simulink model "vf_comparison"  (R2023b)
settings: Solver=VariableStepAuto  StartTime=0.0  StopTime=100  FixedStep=0.001  RelTol=1e-3
undefined symbols (not defined in the file or in its folder): J, K_r, L_m, L_s, R_s, T_r, Z_p
libraries: fuzblock x1, slpidlib x1, rllib x1, dspsrcs4 x1
settings Model: Creator=anste  LastModifiedBy=anste
settings SolverCC: ZeroCrossAlgorithm=Adaptive
settings DebuggingCC: IgnoredZcDiagnostic=none

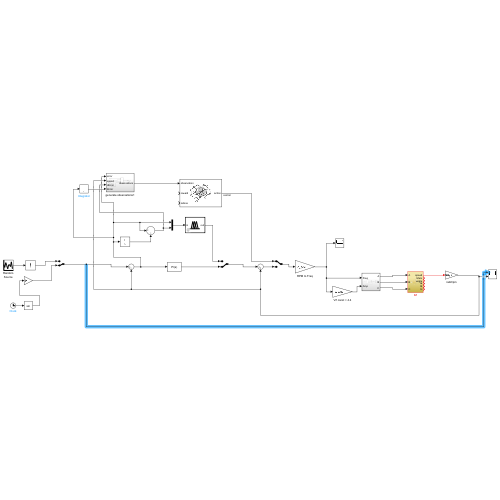
[thumbnail: Simulink's stored preview of the top-level diagram]
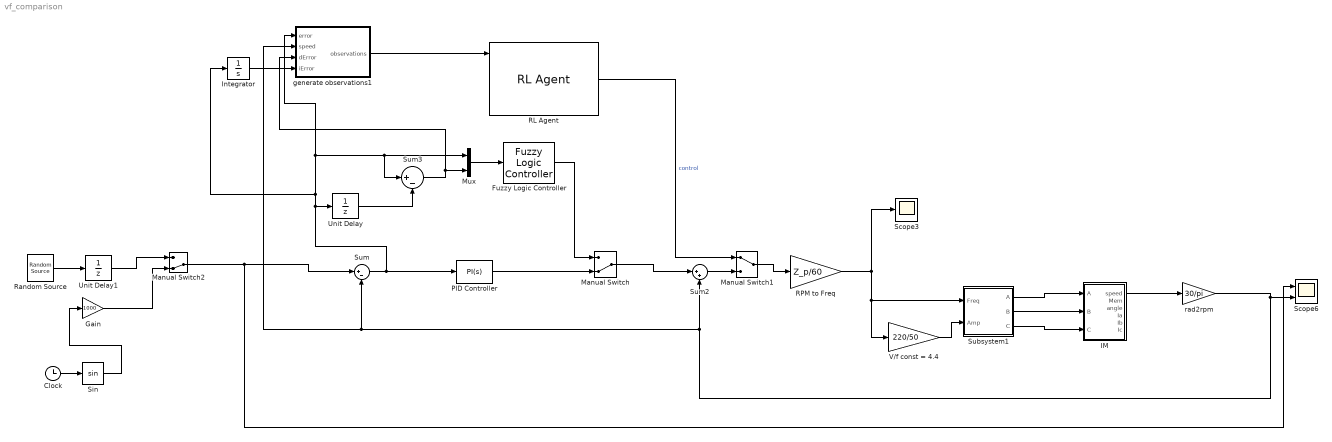
== system vf_comparison ==
  Clock : Clock
  Fuzzy Logic Controller : fuzblock/Fuzzy Logic  Controller  FIS='fuzzy35.fis'  OutputSampleNumber=101  DataType=double  FuzzifiedInputs=off  RuleFiringStrengths=off  RuleOutputs=off  AggregatedOutputs=off  SimulateUsing=Interpreted execution  OutOfRangeInputValueMessage=warning  NoRuleFiredMessage=warning  EmptyOutputFuzzySetMessage=warning
  Gain : Gain  Gain=1000
  IM : Subsystem
  Integrator : Integrator
  Manual Switch : ManualSwitch  CurrentSetting=0
  Manual Switch1 : ManualSwitch
  Manual Switch2 : ManualSwitch  CurrentSetting=0
  Mux : Mux  Inputs=2
  PID Controller : slpidlib/PID Controller  Controller=PI  Form=Parallel  TimeDomain=Continuous-time  UseExternalTs=off  SampleTime=-1  IntegratorMethod=Forward Euler  FilterMethod=Forward Euler  ControllerParametersSource=internal  P=0.42  I=0.87  UseKiTs=off  D=0.000001  N=100  UseFilter=on  TunerSelectOption=Transfer Function Based (PID Tuner App)  InitialConditionSource=internal  InitialConditionForIntegrator=0  InitialConditionForFilter=0  DifferentiatorICPrevScaledInput=0  ExternalReset=none  TrackingMode=off  Kt=1  LimitOutput=off  SatLimitsSource=internal  UpperSaturationLimit=100  LowerSaturationLimit=-100  LinearizeAsGain=on  AntiWindupMode=clamping  Kb=1  LimitIntegrator=off  UpperIntegratorSaturationLimit=inf  LowerIntegratorSaturationLimit=-inf  POutMin=[]  POutMax=[]  IOutMin=[]  IOutMax=[]  DOutMin=[]  DOutMax=[]  NOutMin=[]  NOutMax=[]  SumOutMin=[]  SumOutMax=[]  SaturationOutMin=[]  SaturationOutMax=[]  PParamMin=[]  PParamMax=[]  IParamMin=[]  IParamMax=[]  DParamMin=[]  DParamMax=[]  NParamMin=[]  NParamMax=[]  KbParamMin=[]  KbParamMax=[]  KtParamMin=[]  KtParamMax=[]  KbOutMin=[]  KbOutMax=[]  KtOutMin=[]  KtOutMax=[]  IntegratorOutMin=[]  IntegratorOutMax=[]  FilterOutMin=[]  FilterOutMax=[]  SumI1OutMin=[]  SumI1OutMax=[]  SumI2OutMin=[]  SumI2OutMax=[]  SumI3OutMin=[]  SumI3OutMax=[]  SumI4OutMin=[]  SumI4OutMax=[]  SumDOutMin=[]  SumDOutMax=[]  DifferentiatorOutMin=[]  DifferentiatorOutMax=[]  FilterDiffOutCoefMin=[]  FilterDiffOutCoefMax=[]  ReciprocalOutMin=[]  ReciprocalOutMax=[]  SumDenOutMin=[]  SumDenOutMax=[]  SumNumOutMin=[]  SumNumOutMax=[]  DivideOutMin=[]  DivideOutMax=[]  UdiffTsProdOutMin=[]  UdiffTsProdOutMax=[]  NTsProdOutMin=[]  NTsProdOutMax=[]  UintegralTsProdOutMin=[]  UintegralTsProdOutMax=[]  UngainTsProdOutMin=[]  UngainTsProdOutMax=[]  ClampingZeroOutDataTypeStr=Inherit: Inherit via back propagation  ClampingZeroOutMin=[]  ClampingZeroOutMax=[]  FilterDenConstantOutDataTypeStr=Inherit: Inherit via back propagation  FilterDenConstantOutMin=[]  FilterDenConstantOutMax=[]  PCopyOutDataTypeStr=Inherit: Inherit via back propagation  PCopyOutMin=[]  PCopyOutMax=[]  NCopyOutDataTypeStr=Inherit: Inherit via back propagation  NCopyOutMin=[]  NCopyOutMax=[]  IntegratorContinuousStateAttributes=''  IntegratorStateMustResolveToSignalObject=off  IntegratorRTWStateStorageClass=Auto  FilterContinuousStateAttributes=''  FilterStateMustResolveToSignalObject=off  FilterRTWStateStorageClass=Auto  ParallelPVariant=InternalParameters  IdealPVariant=Disabled  IVariant=InternalParameters  DVariant=Disabled  IntegratorVariant=Continuous  SatVariant=Disabled  AWVariant=Passthrough  PCopyVariant=Disabled  TRVariant=Disabled  FdbkBlocksVariant=Forward  IdealPFdbkVariant=Disabled  SatFdbkVariant=Disabled  DerivativeFilterVariant=Disabled  NVariant=Disabled  NCopyVariant=Disabled_SignalSpec  FilterICVariant=Disabled  IntegratorICVariant=InternalICs  ExternalResetVariant=Disabled  TRSumVariant=Passthrough  SumFdbkVariant=Disabled  SumVariant=Sum_PI  TsampFilterVariant=InternalTs  TsampNgainVariant=Passthrough  TsampIntegralVariant=Disabled_SignalSpec  ExternalSaturationOutDataTypeStr=Inherit: Same as second input
  RL Agent : rllib/RL Agent  Agent=agent  ExternalActionAsInput=off  ProvideLastAction=off  ProvideCumRwd=off  TreatAsDirectFeedthrough=on  UseStrictObservationDataTypes=off
  RPM to Freq : Gain  Gain=Z_p/60
  Random Source : dspsrcs4/Random Source  SrcType=Uniform  NormMethod=Ziggurat  CltLength=12  MinVal=800  MaxVal=1500  MeanVal=0  VarVal=1  RepMode=Specify seed  rawSeed=1  IsInherit=off  SampMode=Discrete  SampTime=1  SampFrame=1  DataType=Double  OutComplex=Real  OutputFrames=off
  Scope3 : Scope
  Scope6 : Scope  NumInputPorts=2
  Sin : Trigonometry
  Subsystem1 : Subsystem
  Sum : Sum  Inputs=|+-
  Sum2 : Sum  Inputs=|++
  Sum3 : Sum  Inputs=|+-
  Unit Delay : UnitDelay  SampleTime=-1
  Unit Delay1 : UnitDelay  SampleTime=3
  V/f const = 4.4 : Gain  Gain=220/50
  generate observations1 : Subsystem
  rad2rpm : Gain  Gain=30/pi
  wires:
  IM/1(speed) -> rad2rpm/1
  rad2rpm/1 -> generate observations1/2(speed), Sum/2, Sum2/2, Scope6/2
  RPM to Freq/1 -> Subsystem1/1(Freq), V/f const = 4.4/1, Scope3/1
  V/f const = 4.4/1 -> Subsystem1/2(Amp)
  Subsystem1/1(A) -> IM/1(A)
  Subsystem1/2(B) -> IM/2(B)
  Subsystem1/3(C) -> IM/3(C)
  Sum/1 -> PID Controller/1, Integrator/1, generate observations1/1(error), Mux/1, Sum3/1, Unit Delay/1
  Sum3/1 -> generate observations1/3(dError), Mux/2
  Unit Delay/1 -> Sum3/2
  Mux/1 -> Fuzzy Logic Controller/1
  Fuzzy Logic Controller/1 -> Manual Switch/1
  PID Controller/1 -> Manual Switch/2
  Manual Switch/1 -> Sum2/1
  Sum2/1 -> Manual Switch1/2
  Manual Switch1/1 -> RPM to Freq/1
  RL Agent/1 -> Manual Switch1/1  "control"
  generate observations1/1(observations) -> RL Agent/1
  Random Source/1 -> Unit Delay1/1
  Integrator/1 -> generate observations1/4(iError)
  Clock/1 -> Sin/1
  Sin/1 -> Gain/1
  Unit Delay1/1 -> Manual Switch2/1
  Gain/1 -> Manual Switch2/2
  Manual Switch2/1 -> Scope6/1, Sum/1

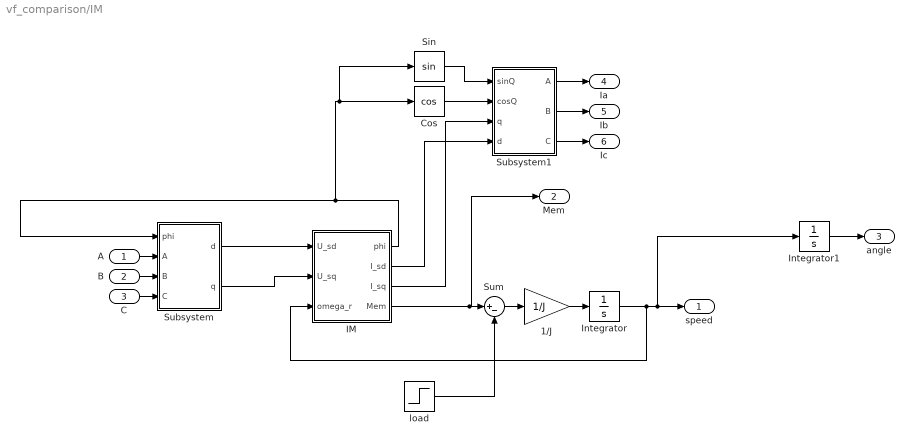
== system vf_comparison/IM ==
  A : Inport
  B : Inport  Port=2
  C : Inport  Port=3
  1/J : Gain  Gain=1/J  SaturateOnIntegerOverflow=on  OutDataTypeStr=Inherit: Same as input  ParamDataTypeStr=Inherit: Same as input
  Cos : Trigonometry  Operator=cos
  IM : Subsystem
  Integrator : Integrator
  Integrator1 : Integrator
  Sin : Trigonometry
  Subsystem : Subsystem
  Subsystem1 : Subsystem
  Sum : Sum  Inputs=|+-
  load : Step  After=0  SampleTime=0
  speed : Outport
  Mem : Outport  Port=2
  angle : Outport  Port=3
  Ia : Outport  Port=4
  Ib : Outport  Port=5
  Ic : Outport  Port=6
  wires:
  B/1 -> Subsystem/3(B)
  Sum/1 -> 1/J/1
  IM/4(Mem) -> Mem/1, Sum/1
  A/1 -> Subsystem/2(A)
  Subsystem/2(q) -> IM/2(U_sq)
  IM/1(phi) -> Sin/1, Cos/1, Subsystem/1(phi)
  Subsystem/1(d) -> IM/1(U_sd)
  1/J/1 -> Integrator/1
  Integrator/1 -> Integrator1/1, speed/1, IM/3(omega_r)
  load/1 -> Sum/2
  C/1 -> Subsystem/4(C)
  Integrator1/1 -> angle/1
  IM/2(I_sd) -> Subsystem1/4(d)
  IM/3(I_sq) -> Subsystem1/3(q)
  Cos/1 -> Subsystem1/2(cosQ)
  Sin/1 -> Subsystem1/1(sinQ)
  Subsystem1/1(A) -> Ia/1
  Subsystem1/2(B) -> Ib/1
  Subsystem1/3(C) -> Ic/1

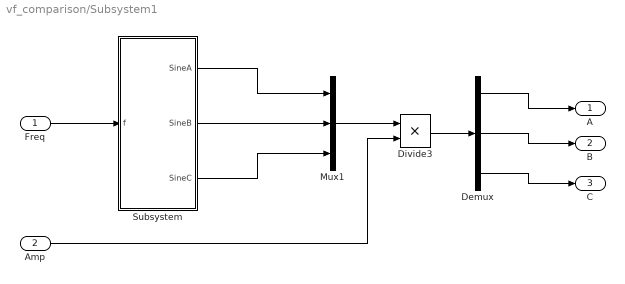
== system vf_comparison/Subsystem1 ==
  Freq : Inport
  Amp : Inport  Port=2
  Demux : Demux  Outputs=3
  Divide3 : Product  Inputs=**
  Mux1 : Mux  Inputs=3
  Subsystem : Subsystem
  A : Outport
  B : Outport  Port=2
  C : Outport  Port=3
  wires:
  Demux/1 -> A/1
  Subsystem/3(SineC) -> Mux1/3
  Divide3/1 -> Demux/1
  Demux/3 -> C/1
  Amp/1 -> Divide3/2
  Subsystem/2(SineB) -> Mux1/2
  Subsystem/1(SineA) -> Mux1/1
  Mux1/1 -> Divide3/1
  Freq/1 -> Subsystem/1(f)
  Demux/2 -> B/1

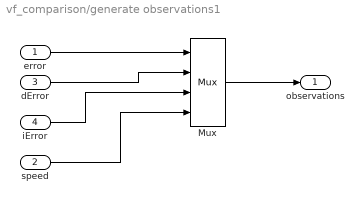
== system vf_comparison/generate observations1 ==
  error : Inport
  speed : Inport  Port=2
  dError : Inport  Port=3
  iError : Inport  Port=4
  Mux : Mux
  observations : Outport  VectorParamsAs1DForOutWhenUnconnected=off
  wires:
  speed/1 -> Mux/4
  Mux/1 -> observations/1
  error/1 -> Mux/1
  dError/1 -> Mux/2
  iError/1 -> Mux/3

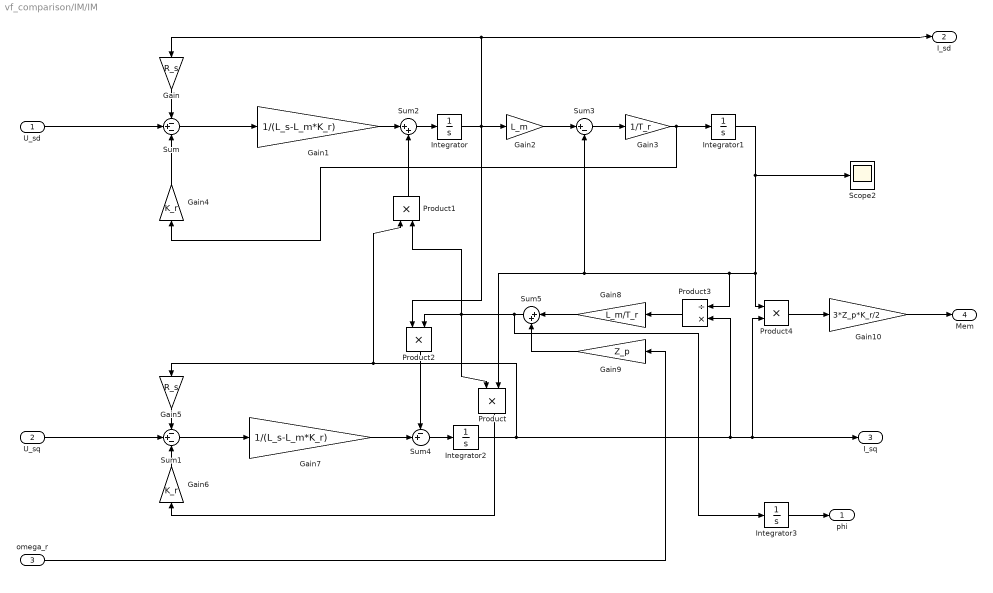
== system vf_comparison/IM/IM ==
  U_sd : Inport
  U_sq : Inport  Port=2
  omega_r : Inport  Port=3
  Gain : Gain  Gain=R_s
  Gain1 : Gain  Gain=1/(L_s-L_m*K_r)
  Gain10 : Gain  Gain=3*Z_p*K_r/2
  Gain2 : Gain  Gain=L_m
  Gain3 : Gain  Gain=1/T_r
  Gain4 : Gain  Gain=K_r
  Gain5 : Gain  Gain=R_s
  Gain6 : Gain  Gain=K_r
  Gain7 : Gain  Gain=1/(L_s-L_m*K_r)
  Gain8 : Gain  Gain=L_m/T_r
  Gain9 : Gain  Gain=Z_p
  Integrator : Integrator
  Integrator1 : Integrator  InitialCondition=1e-10
  Integrator2 : Integrator
  Integrator3 : Integrator
  Product : Product  Inputs=**
  Product1 : Product
  Product2 : Product
  Product3 : Product  Inputs=/*
  Product4 : Product
  Scope2 : Scope
  Sum : Sum  Inputs=-+-
  Sum1 : Sum  Inputs=-+-
  Sum2 : Sum  Inputs=|++
  Sum3 : Sum  Inputs=|+-
  Sum4 : Sum  Inputs=-+|
  Sum5 : Sum  Inputs=|++
  phi : Outport
  I_sd : Outport  Port=2
  I_sq : Outport  Port=3
  Mem : Outport  Port=4
  wires:
  Gain9/1 -> Sum5/2
  Integrator2/1 -> Product3/2, Product4/2, I_sq/1, Product1/1, Gain5/1
  Sum2/1 -> Integrator/1
  Gain2/1 -> Sum3/1
  Sum4/1 -> Integrator2/1
  Sum5/1 -> Integrator3/1, Product/1, Product1/2, Product2/2
  Sum/1 -> Gain1/1
  Sum1/1 -> Gain7/1
  Sum3/1 -> Gain3/1
  Product/1 -> Gain6/1
  Gain/1 -> Sum/1
  Gain7/1 -> Sum4/2
  Gain10/1 -> Mem/1
  Gain3/1 -> Integrator1/1, Gain4/1
  Gain1/1 -> Sum2/1
  Integrator/1 -> Gain2/1, I_sd/1, Gain/1, Product2/1
  Gain4/1 -> Sum/3
  Gain5/1 -> Sum1/1
  Integrator1/1 -> Product4/1, Product3/1, Product/2, Sum3/2, Scope2/1
  Product3/1 -> Gain8/1
  U_sq/1 -> Sum1/2
  Product2/1 -> Sum4/1
  Product4/1 -> Gain10/1
  Product1/1 -> Sum2/2
  Gain8/1 -> Sum5/1
  Gain6/1 -> Sum1/3
  U_sd/1 -> Sum/2
  omega_r/1 -> Gain9/1
  Integrator3/1 -> phi/1

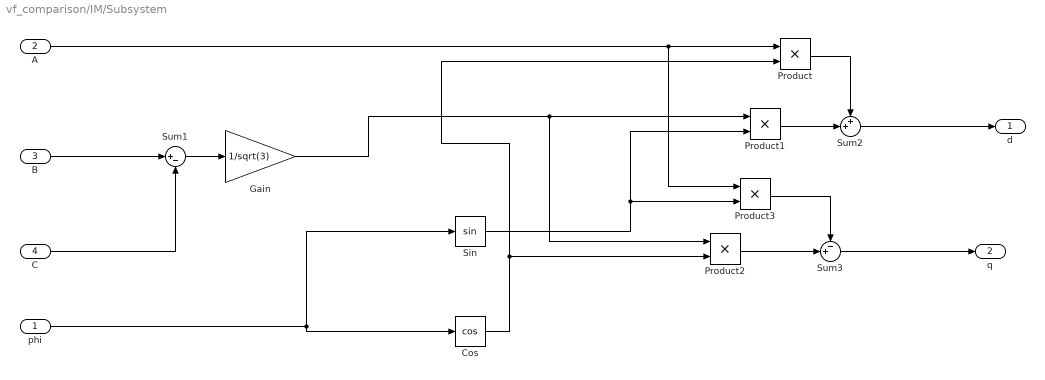
== system vf_comparison/IM/Subsystem ==
  phi : Inport
  A : Inport  Port=2
  B : Inport  Port=3
  C : Inport  Port=4
  Cos : Trigonometry  Operator=cos
  Gain : Gain  Gain=1/sqrt(3)
  Product{,1..3} (4 alike) : Product
  Sin : Trigonometry
  Sum1 : Sum  Inputs=|+-
  Sum2 : Sum  Inputs=++|
  Sum3 : Sum  Inputs=-+|
  d : Outport
  q : Outport  Port=2
  wires:
  phi/1 -> Sin/1, Cos/1
  Sum1/1 -> Gain/1
  Sum2/1 -> d/1
  C/1 -> Sum1/2
  B/1 -> Sum1/1
  Sum3/1 -> q/1
  A/1 -> Product3/1, Product/1
  Cos/1 -> Product2/2, Product/2
  Product/1 -> Sum2/1
  Product1/1 -> Sum2/2
  Gain/1 -> Product2/1, Product1/1
  Sin/1 -> Product3/2, Product1/2
  Product2/1 -> Sum3/2
  Product3/1 -> Sum3/1

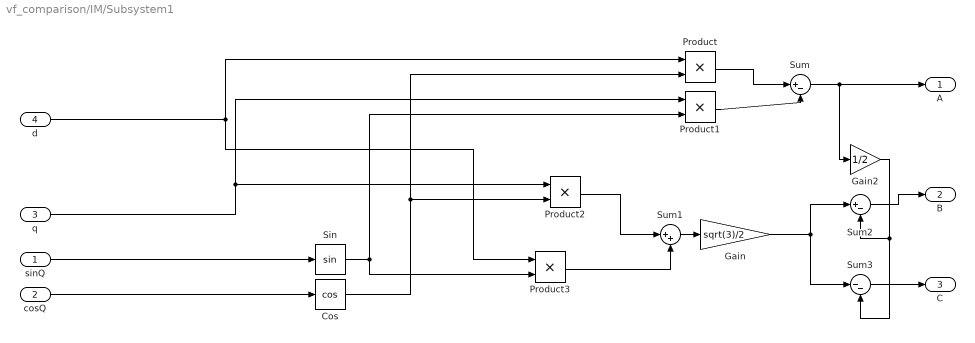
== system vf_comparison/IM/Subsystem1 ==
  sinQ : Inport
  cosQ : Inport  Port=2
  q : Inport  Port=3
  d : Inport  Port=4
  Cos : Trigonometry  Operator=cos
  Gain : Gain  Gain=sqrt(3)/2
  Gain2 : Gain  Gain=1/2
  Product{,1..3} (4 alike) : Product
  Sin : Trigonometry
  Sum : Sum  Inputs=|+-
  Sum1 : Sum  Inputs=|++
  Sum2 : Sum  Inputs=|+-
  Sum3 : Sum  Inputs=|--
  A : Outport
  B : Outport  Port=2
  C : Outport  Port=3
  wires:
  d/1 -> Product/1, Product3/1
  Cos/1 -> Product2/2, Product/2
  Sin/1 -> Product1/2, Product3/2
  q/1 -> Product2/1, Product1/1
  Product/1 -> Sum/1
  Product1/1 -> Sum/2
  Sum/1 -> Gain2/1, A/1
  Product2/1 -> Sum1/1
  Product3/1 -> Sum1/2
  Sum1/1 -> Gain/1
  Sum2/1 -> B/1
  Gain/1 -> Sum3/1, Sum2/1
  Gain2/1 -> Sum3/2, Sum2/2
  Sum3/1 -> C/1
  sinQ/1 -> Sin/1
  cosQ/1 -> Cos/1

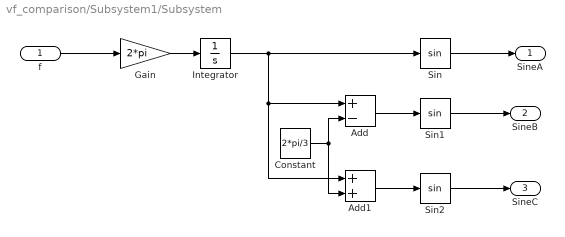
== system vf_comparison/Subsystem1/Subsystem ==
  f : Inport
  Add : Sum  Inputs=+-
  Add1 : Sum
  Constant : Constant  Value=2*pi/3
  Gain : Gain  Gain=2*pi
  Integrator : Integrator
  Sin : Trigonometry
  Sin1 : Trigonometry
  Sin2 : Trigonometry
  SineA : Outport
  SineB : Outport  Port=2
  SineC : Outport  Port=3
  wires:
  Add/1 -> Sin1/1
  Sin/1 -> SineA/1
  Sin1/1 -> SineB/1
  Sin2/1 -> SineC/1
  Constant/1 -> Add1/2, Add/2
  Integrator/1 -> Sin/1, Add/1, Add1/1
  f/1 -> Gain/1
  Add1/1 -> Sin2/1
  Gain/1 -> Integrator/1
